simulink model "KinematicDLQR"  (R2021a)
settings: Solver=FixedStepAuto  StartTime=0.0  StopTime=60  FixedStep=0.01  RelTol=1e-3
values from neighbouring files (symbols this model uses):
  kappar = [kr1,kr2,kr3,kr4,kr5,kr6,kr7,kr8,kr9,kr10,kr11]    [routing_planning.m]
  thetar = [theta1,theta2,theta3,theta4,theta5,theta6,theta7,theta8,theta9,theta10,theta11]    [routing_planning.m]
  vr = 6    [routing_planning.m]
  xr = [x1,x2,x3,x4,x5,x6,x7,x8,x9,x10,x11]    [routing_planning.m]
  yr = [y1,y2,y3,y4,y5,y6,y7,y8,y9,y10,y11]    [routing_planning.m]
libraries: autolibshared x1
settings Model: Creator=xiaochangshui  LastModifiedBy=xiaochangshui

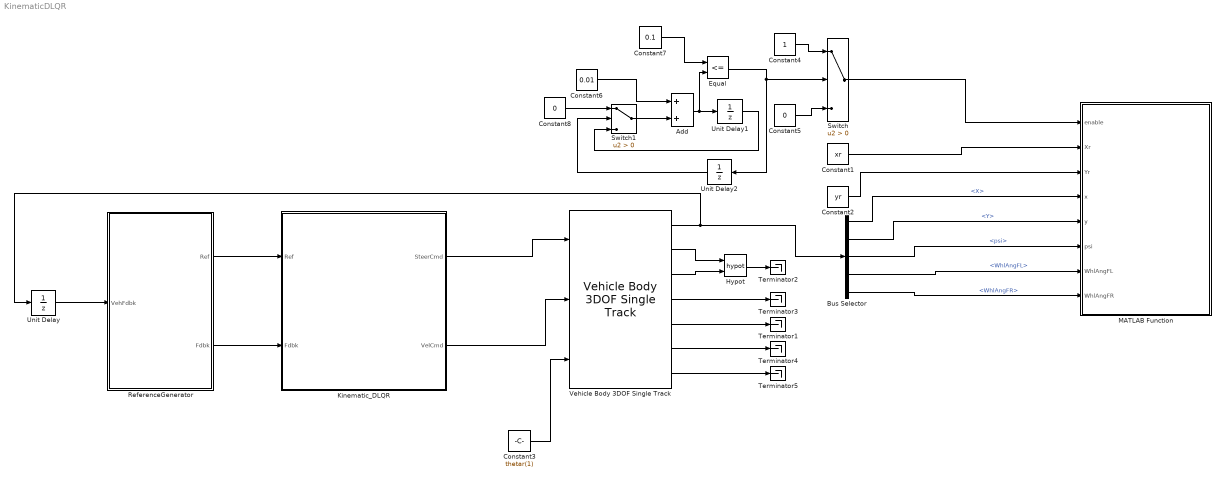
== system KinematicDLQR ==
  Add : Sum
  Bus Selector : BusSelector  OutputSignals=InertFrm.Cg.Disp.X,InertFrm.Cg.Disp.Y,InertFrm.Cg.Ang.psi,BdyFrm.FrntAxl.Steer.WhlAngFL,BdyFrm.FrntAxl.Steer.WhlAngFR
  Constant1 : Constant  Value=xr  SampleTime=-1
  Constant2 : Constant  Value=yr  SampleTime=-1
  Constant3 : Constant  Value=thetar(1)
  Constant4 : Constant
  Constant5 : Constant  Value=0
  Constant6 : Constant  Value=0.01
  Constant7 : Constant  Value=0.1
  Constant8 : Constant  Value=0
  Equal : RelationalOperator  Operator=<=  OutDataTypeStr=boolean  RndMeth=Simplest
  Hypot : Math  Operator=hypot  SaturateOnIntegerOverflow=on
  Kinematic_DLQR : Subsystem  VariantControl=(default)
      mask Display: image('LongitudinalDriver.png'); % Use "Edit Image" on toolstrip to change.
  MATLAB Function : MATLAB Function  TreatAsAtomicUnit=on
  ReferenceGenerator : Subsystem
  Switch : Switch  Criteria=u2 > Threshold
  Switch1 : Switch  Criteria=u2 > Threshold
  Terminator{1..5} (5 alike) : Terminator
  Unit Delay : UnitDelay  SampleTime=-1  HasFrameUpgradeWarning=on
  Unit Delay1 : UnitDelay  SampleTime=-1  HasFrameUpgradeWarning=on
  Unit Delay2 : UnitDelay  SampleTime=-1  HasFrameUpgradeWarning=on
  Vehicle Body 3DOF Single Track : autolibshared/Vehicle Body 3DOF Single Track  trackMode=Single (bicycle)  inputMode=External longitudinal velocity  frontSteerMode=on  rearSteerMode=off  windMode=off  muMode=off  extFMode=off  extMMode=off  htchFMode=off  htchMMode=off  extXo=off  extpsio=on  extxdoto=off  extro=off  extYo=off  extTamb=off  extydoto=off  aMode=2  NF=2  NR=2  m=2000  a=1.4  b=1.6  h=0.35  dh=1  hh=0.2  X_o=0  xdot_o=0  CalphaMode=off  sigmaMode=on  d=0  hl=0  w=[1.4,1.4]  Cy_f=12e3  Cy_r=11e3  sigma_f=.1  sigma_r=.1  alpha_f_brk=[-.1 .1]  Cy_f_data=[-9e3 9e3]  alpha_r_brk=[-.1 .1]  Cy_r_data=[-9e3 9e3]  Y_o=0  ydot_o=0  Izz=4000  psi_o=0  r_o=0  Af=2  Cd=.3  Cl=.1  Cpm=.1  beta_w=[0:0.01:0.3]  Cs=[0:0.03:0.9]  Cym=[0:0.01:0.3]  Pabs=101325  Tair=273  g=9.81  mu=1  xdot_tol=.01  Fznom=5000  Fxtire_sat=7e4  Fytire_sat=7e4  longOff=0  latOff=0  vertOff=0  wrapAng=off
      settings: SourceProductBaseCode=PW,DR,MT,UV,VE
  wires:
  Vehicle Body 3DOF Single Track/4 -> Terminator3/1
  Vehicle Body 3DOF Single Track/3 -> Hypot/2
  Vehicle Body 3DOF Single Track/1 -> Bus Selector/1, Unit Delay/1
  Vehicle Body 3DOF Single Track/2 -> Hypot/1
  ReferenceGenerator/1(Ref) -> Kinematic_DLQR/1(Ref)
  ReferenceGenerator/2(Fdbk) -> Kinematic_DLQR/2(Fdbk)
  Hypot/1 -> Terminator2/1
  Vehicle Body 3DOF Single Track/5 -> Terminator1/1
  Vehicle Body 3DOF Single Track/6 -> Terminator4/1
  Vehicle Body 3DOF Single Track/7 -> Terminator5/1
  Unit Delay/1 -> ReferenceGenerator/1(VehFdbk)
  Kinematic_DLQR/2(VelCmd) -> Vehicle Body 3DOF Single Track/2
  Kinematic_DLQR/1(SteerCmd) -> Vehicle Body 3DOF Single Track/1
  Constant1/1 -> MATLAB Function/2(Xr)
  Constant2/1 -> MATLAB Function/3(Yr)
  Bus Selector/1 -> MATLAB Function/4(x)  "<X>"
  Bus Selector/2 -> MATLAB Function/5(y)  "<Y>"
  Bus Selector/3 -> MATLAB Function/6(psi)  "<psi>"
  Bus Selector/4 -> MATLAB Function/7(WhlAngFL)  "<WhlAngFL>"
  Bus Selector/5 -> MATLAB Function/8(WhlAngFR)  "<WhlAngFR>"
  Switch/1 -> MATLAB Function/1(enable)
  Constant3/1 -> Vehicle Body 3DOF Single Track/3
  Constant8/1 -> Switch1/1
  Unit Delay2/1 -> Switch1/2
  Switch1/1 -> Add/2
  Unit Delay1/1 -> Switch1/3
  Constant7/1 -> Equal/1
  Add/1 -> Equal/2, Unit Delay1/1
  Equal/1 -> Unit Delay2/1, Switch/2
  Constant5/1 -> Switch/3
  Constant4/1 -> Switch/1
  Constant6/1 -> Add/1

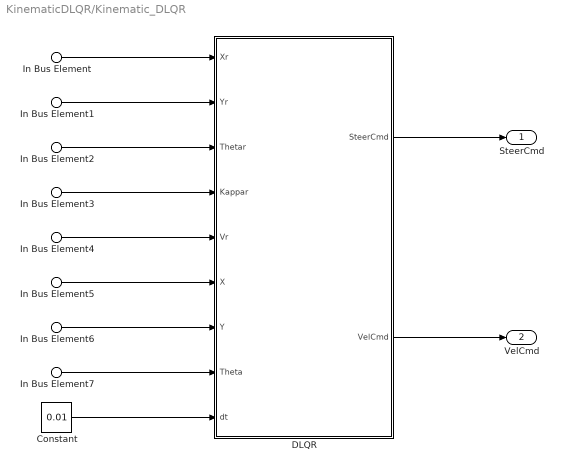
== system KinematicDLQR/Kinematic_DLQR ==
  In Bus Element : Inport  PortName=Ref  Element=X
  In Bus Element1 : Inport  PortName=Ref  Element=Y
  In Bus Element2 : Inport  PortName=Ref  Element=Theta
  In Bus Element3 : Inport  PortName=Ref  Element=Kappa
  In Bus Element4 : Inport  PortName=Ref  Element=V
  In Bus Element5 : Inport  Port=2  PortName=Fdbk  Element=InertFrm.Cg.Disp.X
  In Bus Element6 : Inport  Port=2  PortName=Fdbk  Element=InertFrm.Cg.Disp.Y
  In Bus Element7 : Inport  Port=2  PortName=Fdbk  Element=InertFrm.Cg.Ang.psi
  Constant : Constant  Value=0.01
  DLQR : MATLAB Function  TreatAsAtomicUnit=on
  SteerCmd : Outport
  VelCmd : Outport  Port=2
  wires:
  DLQR/1(SteerCmd) -> SteerCmd/1
  DLQR/2(VelCmd) -> VelCmd/1
  Constant/1 -> DLQR/9(dt)
  In Bus Element/1 -> DLQR/1(Xr)
  In Bus Element1/1 -> DLQR/2(Yr)
  In Bus Element2/1 -> DLQR/3(Thetar)
  In Bus Element3/1 -> DLQR/4(Kappar)
  In Bus Element4/1 -> DLQR/5(Vr)
  In Bus Element5/1 -> DLQR/6(X)
  In Bus Element7/1 -> DLQR/8(Theta)
  In Bus Element6/1 -> DLQR/7(Y)

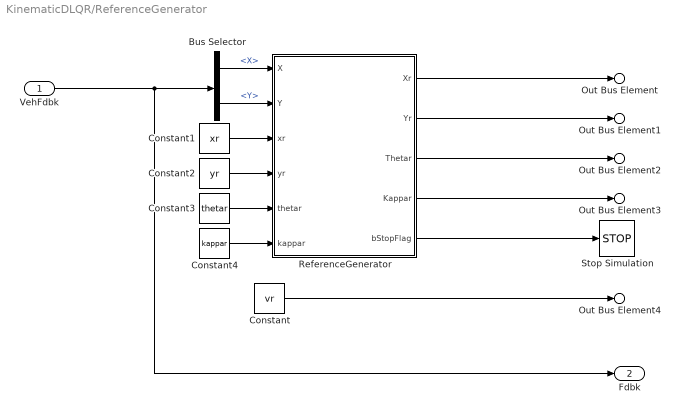
== system KinematicDLQR/ReferenceGenerator ==
  VehFdbk : Inport
  Bus Selector : BusSelector  OutputSignals=InertFrm.Cg.Disp.X,InertFrm.Cg.Disp.Y
  Constant : Constant  Value=vr  SampleTime=-1
  Constant1 : Constant  Value=xr  SampleTime=-1
  Constant2 : Constant  Value=yr  SampleTime=-1
  Constant3 : Constant  Value=thetar  SampleTime=-1
  Constant4 : Constant  Value=kappar  SampleTime=-1
  ReferenceGenerator : MATLAB Function  TreatAsAtomicUnit=on  VariantControl=Choice
  Stop Simulation : Stop
  Out Bus Element : Outport  PortName=Ref  Element=X
  Out Bus Element1 : Outport  PortName=Ref  Element=Y
  Out Bus Element2 : Outport  PortName=Ref  Element=Theta
  Out Bus Element3 : Outport  PortName=Ref  Element=Kappa
  Out Bus Element4 : Outport  PortName=Ref  Element=V
  Fdbk : Outport  Port=2
  wires:
  Bus Selector/1 -> ReferenceGenerator/1(X)  "<X>"
  Bus Selector/2 -> ReferenceGenerator/2(Y)  "<Y>"
  ReferenceGenerator/1(Xr) -> Out Bus Element/1
  ReferenceGenerator/2(Yr) -> Out Bus Element1/1
  ReferenceGenerator/3(Thetar) -> Out Bus Element2/1
  ReferenceGenerator/4(Kappar) -> Out Bus Element3/1
  Constant/1 -> Out Bus Element4/1
  Constant1/1 -> ReferenceGenerator/3(xr)
  Constant2/1 -> ReferenceGenerator/4(yr)
  Constant3/1 -> ReferenceGenerator/5(thetar)
  Constant4/1 -> ReferenceGenerator/6(kappar)
  VehFdbk/1 -> Fdbk/1, Bus Selector/1
  ReferenceGenerator/5(bStopFlag) -> Stop Simulation/1

== matlab function KinematicDLQR/MATLAB Function ==
  data: enable input; Xr input; Yr input; x input; y input; psi input; WhlAngFL input; WhlAngFR input
function fcn(enable, Xr, Yr, x, y, psi, WhlAngFL, WhlAngFR)
    
    if ~enable
        return;
    end
    figure(1)
    clf;
    axis equal;
    hold on;grid on;
    plot(Xr, Yr, 'r', 'LineWidth', 2)
    veh.LB = 2.7;
    veh.LF = 0.95;
    veh.LR = 1.05;
    veh.W = 1.8;
    veh.WR = 0.3;
    xlim(x + [-10, 10])
    ylim(y + [-10, 10])
    
    R = [cos(psi), -sin(psi); sin(psi), cos(psi)]; 
    FL = [x; y] + R * [veh.LB + veh.LF; 0.5 * veh.W];
    FR = [x; y] + R * [veh.LB + veh.LF; -0.5 * veh.W];
    RL = [x; y] + R * [-veh.LR; 0.5 * veh.W];
    RR = [x; y] + R * [-veh.LR; -0.5 * veh.W];
    
    vehx = [FL(1),FR(1),RR(1),RL(1),FL(1)];
    vehy = [FL(2),FR(2),RR(2),RL(2),FL(2)];
    plot(vehx, vehy, 'b', 'LineWidth', 0.5);
    
    FAC = [x; y] + R * [veh.LB; 0.0];
    plot([x, FAC(1)], [y, FAC(2)], 'k', 'LineWidth', 3)
    
    RAL = [x; y] + R * [0.0; 0.5 * veh.W - 0.2];
    RAR = [x; y] + R * [0.0; -0.5 * veh.W + 0.2];
    plot([RAL(1), RAR(1)], [RAL(2), RAR(2)], 'k', 'LineWidth', 3)
    
    FAL = [x; y] + R * [veh.LB; 0.5 * veh.W - 0.2];
    FAR = [x; y] + R * [veh.LB; -0.5 * veh.W + 0.2];
    plot([FAL(1), FAR(1)], [FAL(2), FAR(2)], 'k', 'LineWidth', 3)
    
    RWL1 = [x; y] + R * [veh.WR; 0.5 * veh.W - 0.2];
    RWL2 = [x; y] + R * [-veh.WR; 0.5 * veh.W - 0.2];
    plot([RWL1(1), RWL2(1)], [RWL1(2), RWL2(2)], 'k', 'LineWidth', 3)
    
    RWR1 = [x; y] + R * [veh.WR; -0.5 * veh.W + 0.2];
    RWR2 = [x; y] + R * [-veh.WR; -0.5 * veh.W + 0.2];
    plot([RWR1(1), RWR2(1)], [RWR1(2), RWR2(2)], 'k', 'LineWidth', 3)
    
    FWL1 = [x; y] + R * ([veh.LB; 0.5 * veh.W - 0.2] + veh.WR * [cos(WhlAngFL); sin(WhlAngFL)]);
    FWL2 = [x; y] + R * ([veh.LB; 0.5 * veh.W - 0.2] - veh.WR * [cos(WhlAngFL); sin(WhlAngFL)]);
    plot([FWL1(1), FWL2(1)], [FWL1(2), FWL2(2)], 'k', 'LineWidth', 3)
    
    FWR1 = [x; y] + R * ([veh.LB; -0.5 * veh.W + 0.2] + veh.WR * [cos(WhlAngFR); sin(WhlAngFR)]);
    FWR2 = [x; y] + R * ([veh.LB; -0.5 * veh.W + 0.2] - veh.WR * [cos(WhlAngFR); sin(WhlAngFR)]);
    plot([FWR1(1), FWR2(1)], [FWR1(2), FWR2(2)], 'k', 'LineWidth', 3)
    
    plot(x, y, 'cp') 
end

== matlab function KinematicDLQR/Kinematic_DLQR/DLQR ==
  data: Xr input; Yr input; Thetar input; Kappar input; Vr input; X input; Y input; Theta input; SteerCmd output; VelCmd output; dt input
function [SteerCmd, VelCmd] = DLQR(Xr, Yr, Thetar, Kappar, Vr, X, Y, Theta, dt)
    
%     coder.extrinsic('dlqr');
%     K = zeros(2, 3);
    L = 1.6;
    
    Q = [5, 0, 0;
          0, 5, 0;
          0, 0, 50];
      
    R = [1, 0;
          0, 1];
    
    A = [1, 0, -Vr * sin(Thetar) * dt;
        0, 1, Vr * cos(Thetar) * dt;
        0, 0, 1];
    
    B = [cos(Thetar) * dt, 0;
        sin(Thetar) * dt, 0;
        Kappar * dt, Vr / L / cos(Thetar) ^ 2 * dt];
    
    dX = X - Xr;
    dY = Y - Yr;
    dTheta = Theta - Thetar;
    if dTheta > pi
        dTheta = dTheta - 2 * pi;
    elseif dTheta < -pi
        dTheta = dTheta + 2 * pi;
    end
    
    S = [dX; dY; dTheta];
    
    P_1 = Q;
    for i = 1 : 100
       K = (R + B' * P_1 * B) \ (B' * P_1 * A);
       P = Q + A' * P_1 * A - A' * P_1 * B * K;
       if norm(P - P_1) < 0.1
           break;
       else
           P_1 = P;
       end
    end
%     K = dlqr(A, B, Q, R);
    U = -K * S;
%     U = -K * S;
    SteerCmd = atan(L * Kappar) + U(2);
    VelCmd = Vr + U(1);
end

== matlab function KinematicDLQR/ReferenceGenerator/ReferenceGenerator ==
  settings: updateMethod=DISCRETE
  data: Xr output; X input; Y input; Yr output; Thetar output; Kappar output; xr input; yr input; thetar input; kappar input; bStopFlag output
function [Xr, Yr, Thetar, Kappar, bStopFlag] = ReferenceGenerator(X, Y, xr, yr, thetar, kappar)

    persistent start_index
    if isempty(start_index)
        start_index = uint32(1);
    end

    min_dist = 1000;
    for idx = start_index : min(start_index + 30, length(xr))
        dist = distance(X, Y, xr(idx), yr(idx));
        if dist < min_dist
            min_dist = dist;
            start_index = idx;
        end
    end
    if min_index == length(xr)
        bStopFlag = true;
    else
        bStopFlag = false;
    end
    Xr = xr(start_index);
    Yr = yr(start_index);
    Thetar = thetar(start_index);
    Kappar = kappar(start_index);
end

function dist = distance(x1, y1, x2, y2)
   dist = sqrt((x2 - x1) ^ 2 + (y2 - y1) ^ 2); 
end
